simulink model "FirstNonLinearModel"  (R2020b)
settings: Solver=VariableStepAuto  StartTime=0.0  StopTime=1000  RelTol=1e-3
settings Model: Creator=karshenas  LastModifiedBy=karshenas

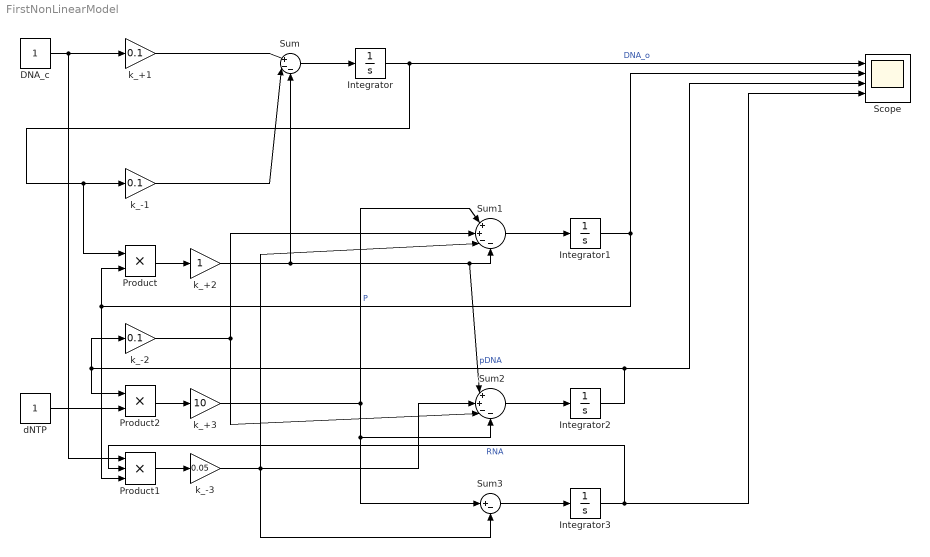
== system FirstNonLinearModel ==
  DNA_c : Constant
  Integrator{,1..3} (4 alike) : Integrator
  Product : Product
  Product1 : Product  Inputs=3
  Product2 : Product
  Scope : Scope  NumInputPorts=4
  Sum : Sum  Inputs=|+--
  Sum1 : Sum  Inputs=|++--
  Sum2 : Sum  Inputs=|++--
  Sum3 : Sum  Inputs=|+-
  dNTP : Constant
  k_+1 : Gain  Gain=0.1
  k_+2 : Gain
  k_+3 : Gain  Gain=10
  k_-1 : Gain  Gain=0.1
  k_-2 : Gain  Gain=0.1
  k_-3 : Gain  Gain=0.05
  wires:
  DNA_c/1 -> Product1/1, k_+1/1
  Sum/1 -> Integrator/1
  Integrator/1 -> Scope/1, Product/1, k_-1/1  "DNA_o"
  k_+1/1 -> Sum/1
  k_-1/1 -> Sum/2
  Product/1 -> k_+2/1
  k_+2/1 -> Sum2/1, Sum1/4, Sum/3
  Integrator1/1 -> Scope/2, Product/2, Product1/3  "P"
  Sum1/1 -> Integrator1/1
  dNTP/1 -> Product2/2
  k_-2/1 -> Sum2/3, Sum1/2
  Integrator2/1 -> Product2/1, k_-2/1, Scope/3  "pDNA"
  Product2/1 -> k_+3/1
  k_+3/1 -> Sum3/1, Sum2/4, Sum1/1
  Integrator3/1 -> Product1/2, Scope/4  "RNA"
  Product1/1 -> k_-3/1
  k_-3/1 -> Sum3/2, Sum2/2, Sum1/3
  Sum2/1 -> Integrator2/1
  Sum3/1 -> Integrator3/1
